simulink model "q4"  (R2017a)
settings: Solver=VariableStepAuto  StartTime=0.0  StopTime=10.0  RelTol=1e-3
values from neighbouring files (symbols this model uses):
  C = [1 0]    [workspace.m]
  F = [f1 f2]    [workspace.m]
  fa = -0.35*f2 + 4.45    (= 3.125)    [workspace.m]
  G = [[0.5 1]; [0.5 0.7]]    [workspace.m]
  H1 = [0.2; 0.1]    [workspace.m]
  H2 = [1; 0]    [workspace.m]
  L = [l1; l2]    [workspace.m]
settings Model: Creator=arthur  LastModifiedBy=arthur

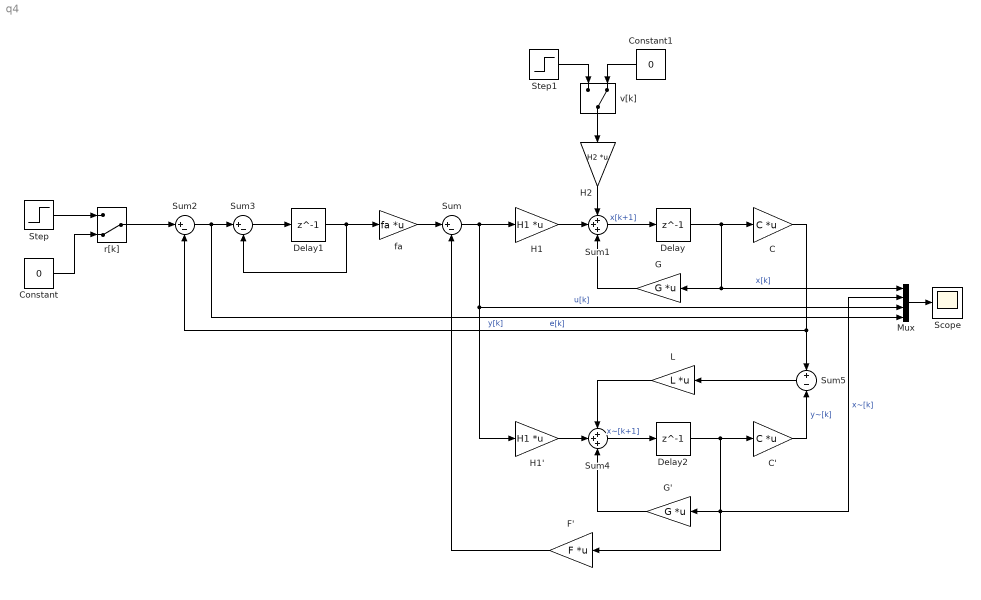
== system q4 ==
  C : Gain  Gain=C  Multiplication=Matrix(K*u)
  C' : Gain  Gain=C  Multiplication=Matrix(K*u)
  Constant : Constant  Value=0
  Constant1 : Constant  Value=0
  Delay : Delay  DelayLength=1  InitialCondition=[1; -1]
  Delay1 : Delay  DelayLength=1  InitialCondition=0
  Delay2 : Delay  DelayLength=1  InitialCondition=0
  F' : Gain  Gain=F  Multiplication=Matrix(K*u)
  G : Gain  Gain=G  Multiplication=Matrix(K*u)
  G' : Gain  Gain=G  Multiplication=Matrix(K*u)
  H1 : Gain  Gain=H1  Multiplication=Matrix(K*u)
  H1' : Gain  Gain=H1  Multiplication=Matrix(K*u)
  H2 : Gain  Gain=H2  Multiplication=Matrix(K*u)
  L : Gain  Gain=L  Multiplication=Matrix(K*u)
  Mux : Mux
  Scope : Scope
  Step : Step  Time=0  SampleTime=0
  Step1 : Step  Time=0  SampleTime=0
  Sum : Sum  Inputs=|+-
  Sum1 : Sum  Inputs=+++
  Sum2 : Sum  Inputs=|+-
  Sum3 : Sum  Inputs=|+-
  Sum4 : Sum  Inputs=+++
  Sum5 : Sum  Inputs=+|-
  fa : Gain  Gain=fa  Multiplication=Matrix(K*u)
  r[k] : ManualSwitch  CurrentSetting=0
  v[k] : ManualSwitch  CurrentSetting=0
  wires:
  r[k]/1 -> Sum2/1
  Sum2/1 -> Mux/4, Sum3/1  "e[k]"
  Sum3/1 -> Delay1/1
  Delay1/1 -> fa/1, Sum3/2
  fa/1 -> Sum/1
  Sum/1 -> H1'/1, Mux/3, H1/1  "u[k]"
  H2/1 -> Sum1/1
  H1/1 -> Sum1/2
  v[k]/1 -> H2/1
  Sum1/1 -> Delay/1  "x[k+1]"
  Delay/1 -> Mux/1, G/1, C/1  "x[k]"
  G/1 -> Sum1/3
  C/1 -> Sum2/2, Sum5/1  "y[k]"
  Step1/1 -> v[k]/1
  Step/1 -> r[k]/1
  Constant/1 -> r[k]/2
  Constant1/1 -> v[k]/2
  H1'/1 -> Sum4/2
  Sum4/1 -> Delay2/1  "x~[k+1]"
  Delay2/1 -> Mux/2, F'/1, G'/1, C'/1  "x~[k]"
  G'/1 -> Sum4/3
  F'/1 -> Sum/2
  C'/1 -> Sum5/2  "y~[k]"
  Sum5/1 -> L/1
  L/1 -> Sum4/1
  Mux/1 -> Scope/1
